simulink model "FCW_a1"  (Simulink 8.7)
settings: Solver=ode1  SolverMode=SingleTasking  StartTime=0.0  StopTime=500  FixedStep=0.001  RelTol=1e-3
(part 2 of 4)

== system FCW_a1/Veh_1_1/DriverModel ==
  note: Help
  VehicleInput : Inport
  Bus Creator37 : BusCreator  Inputs=10
  Bus Creator38 : BusCreator  Inputs=2
  Bus Creator39 : BusCreator  Inputs=2
  Bus Creator6 : BusCreator  Inputs=4
  Bus Selector : BusSelector  OutputSignals=Body_Out_Bus,Steer_Out_Bus,Power_Out_BUs,Brake_Out_Bus
  Bus Selector29 : BusSelector  OutputSignals=Chassi_States.q0,Chassi_States.q1,Chassi_States.q3,Chassi_States.u0,Chassi_States.u1,Chassi_States.u3,Wheel_LF.u1,Wheel_RF.u1,Wheel_LR.u1,Wheel_RR.u1
  Bus Selector30 : BusSelector  OutputSignals=Steer_Kinematics.str_sus_f,Steer_Kinematics.str_sus_r
  Bus Selector31 : BusSelector  OutputSignals=Powertrain_Output.av_eng,Powertrain_Output.aa_eng
  Bus Selector32 : BusSelector  OutputSignals=Brake_Output.turn_off
  Driver : Subsystem
  DriverOut : Outport
  wires:
  Bus Creator6/1 -> DriverOut/1  "Driver_Bus"
  Bus Creator39/1 -> Driver/3(Engine Input)
  Bus Selector31/2 -> Bus Creator39/2  "<aa_eng>"
  Bus Selector31/1 -> Bus Creator39/1  "<av_eng>"
  Bus Selector/3 -> Bus Selector31/1  "<Power_Out_BUs>"
  Bus Selector32/1 -> Driver/4(Brake Input)  "<turn_off>"
  Bus Creator38/1 -> Driver/2(Steer Input)
  Bus Selector30/2 -> Bus Creator38/2  "<str_sus_r>"
  Bus Selector30/1 -> Bus Creator38/1  "<str_sus_f>"
  Bus Selector/2 -> Bus Selector30/1  "<Steer_Out_Bus>"
  Bus Selector29/10 -> Bus Creator37/10  "<u1>"
  Bus Selector29/9 -> Bus Creator37/9  "<u1>"
  Bus Selector29/8 -> Bus Creator37/8  "<u1>"
  Bus Selector29/7 -> Bus Creator37/7  "<u1>"
  Bus Selector29/6 -> Bus Creator37/6  "<u3>"
  Bus Selector29/5 -> Bus Creator37/5  "<u1>"
  Bus Selector29/4 -> Bus Creator37/4  "<u0>"
  Bus Selector29/3 -> Bus Creator37/3  "<q3>"
  Bus Selector29/2 -> Bus Creator37/2  "<q1>"
  Bus Selector29/1 -> Bus Creator37/1  "<q0>"
  Bus Creator37/1 -> Driver/1(Body Input)
  Bus Selector/1 -> Bus Selector29/1  "<Body_Out_Bus>"
  Driver/4(Driver_Brake) -> Bus Creator6/4
  Driver/3(Driver_Powertrain) -> Bus Creator6/3
  Driver/2(Driver_Steer) -> Bus Creator6/2
  Driver/1(Driver_States) -> Bus Creator6/1
  VehicleInput/1 -> Bus Selector/1
  Bus Selector/4 -> Bus Selector32/1  "<Brake_Out_Bus>"

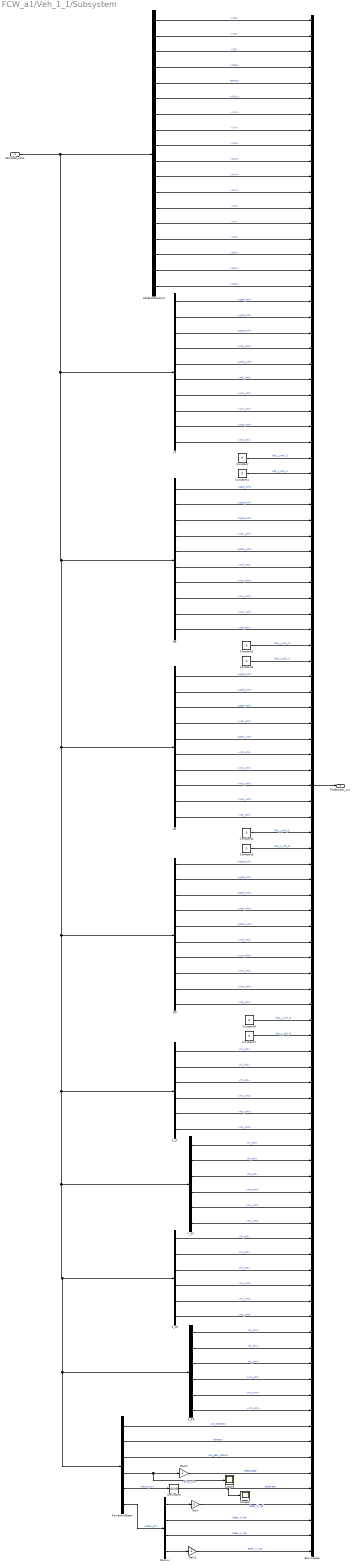
== system FCW_a1/Veh_1_1/Subsystem ==
  VehicleDynOut : Inport
  Bus Creator : BusCreator  Inputs=99
  Constant{,1..7} (8 alike) : Constant  Value=0
  Demux : Demux
  Derivative : Derivative
  F_LF : BusSelector  Tag=PanoSim_System  OutputSignals=Body_Out_Bus.Wheel_LF.fx_whl,Body_Out_Bus.Wheel_LF.fy_whl,Body_Out_Bus.Wheel_LF.fz_whl,Body_Out_Bus.Wheel_LF.mx_whl,Body_Out_Bus.Wheel_LF.my_whl,Body_Out_Bus.Wheel_LF.mz_whl
  F_LR : BusSelector  Tag=PanoSim_System  OutputSignals=Body_Out_Bus.Wheel_LR.fx_whl,Body_Out_Bus.Wheel_LR.fy_whl,Body_Out_Bus.Wheel_LR.fz_whl,Body_Out_Bus.Wheel_LR.mx_whl,Body_Out_Bus.Wheel_LR.my_whl,Body_Out_Bus.Wheel_LR.mz_whl
  F_RF : BusSelector  Tag=PanoSim_System  OutputSignals=Body_Out_Bus.Wheel_RF.fx_whl,Body_Out_Bus.Wheel_RF.fy_whl,Body_Out_Bus.Wheel_RF.fz_whl,Body_Out_Bus.Wheel_RF.mx_whl,Body_Out_Bus.Wheel_RF.my_whl,Body_Out_Bus.Wheel_RF.mz_whl
  F_RR : BusSelector  Tag=PanoSim_System  OutputSignals=Body_Out_Bus.Wheel_RR.fx_whl,Body_Out_Bus.Wheel_RR.fy_whl,Body_Out_Bus.Wheel_RR.fz_whl,Body_Out_Bus.Wheel_RR.mx_whl,Body_Out_Bus.Wheel_RR.my_whl,Body_Out_Bus.Wheel_RR.mz_whl
  Gain : Gain  Gain=-1
  Gain1 : Gain  Gain=-1
  Gain2 : Gain
  LF : BusSelector  Tag=PanoSim_System  OutputSignals=BodyKin_Wheel_Out_Bus.bodykin_whl_out_lf.xgnd_whl,BodyKin_Wheel_Out_Bus.bodykin_whl_out_lf.ygnd_whl,BodyKin_Wheel_Out_Bus.bodykin_whl_out_lf.zgnd_whl,BodyKin_Wheel_Out_Bus.bodykin_whl_out_lf.yaw_whl,BodyKin_Wheel_Out_Bus.bodykin_whl_out_lf.pitch_whl,BodyKin_Wheel_Out_Bus.bodykin_whl_out_lf.roll_whl,BodyKin_Wheel_Out_Bus.bodykin_whl_out_lf.vwx_whl,BodyKin_Wheel_Out_Bus.bodykin_whl_out_lf.vwy_whl,BodyKin_Wheel_Out_Bus.bodykin_whl_out_lf.vwz_whl,BodyKin_Wheel_Out_Bus.bodykin_whl_out_lf.rot_whl
  LR : BusSelector  Tag=PanoSim_System  OutputSignals=BodyKin_Wheel_Out_Bus.bodykin_whl_out_lr.xgnd_whl,BodyKin_Wheel_Out_Bus.bodykin_whl_out_lr.ygnd_whl,BodyKin_Wheel_Out_Bus.bodykin_whl_out_lr.zgnd_whl,BodyKin_Wheel_Out_Bus.bodykin_whl_out_lr.yaw_whl,BodyKin_Wheel_Out_Bus.bodykin_whl_out_lr.pitch_whl,BodyKin_Wheel_Out_Bus.bodykin_whl_out_lr.roll_whl,BodyKin_Wheel_Out_Bus.bodykin_whl_out_lr.vwx_whl,BodyKin_Wheel_Out_Bus.bodykin_whl_out_lr.vwy_whl,BodyKin_Wheel_Out_Bus.bodykin_whl_out_lr.vwz_whl,BodyKin_Wheel_Out_Bus.bodykin_whl_out_lr.rot_whl
  PowerandSteer : BusSelector  Tag=PanoSim_System  OutputSignals=Power_Out_BUs.Powertrain_Output.pt_throttle,Brake_Out_Bus.Brake_Output.brake,Power_Out_BUs.Powertrain_Output.pt_gear_status,Steer_Out_Bus.Steer_Kinematics.strav_sw,Steer_Out_Bus.Steer_Kinematics.strav_sw,Steer_Out_Bus.Steer_Kinematics.steer_str
  RF : BusSelector  Tag=PanoSim_System  OutputSignals=BodyKin_Wheel_Out_Bus.bodykin_whl_out_rf.xgnd_whl,BodyKin_Wheel_Out_Bus.bodykin_whl_out_rf.ygnd_whl,BodyKin_Wheel_Out_Bus.bodykin_whl_out_rf.zgnd_whl,BodyKin_Wheel_Out_Bus.bodykin_whl_out_rf.yaw_whl,BodyKin_Wheel_Out_Bus.bodykin_whl_out_rf.pitch_whl,BodyKin_Wheel_Out_Bus.bodykin_whl_out_rf.roll_whl,BodyKin_Wheel_Out_Bus.bodykin_whl_out_rf.vwx_whl,BodyKin_Wheel_Out_Bus.bodykin_whl_out_rf.vwy_whl,BodyKin_Wheel_Out_Bus.bodykin_whl_out_rf.vwz_whl,BodyKin_Wheel_Out_Bus.bodykin_whl_out_rf.rot_whl
  RR : BusSelector  Tag=PanoSim_System  OutputSignals=BodyKin_Wheel_Out_Bus.bodykin_whl_out_rr.xgnd_whl,BodyKin_Wheel_Out_Bus.bodykin_whl_out_rr.ygnd_whl,BodyKin_Wheel_Out_Bus.bodykin_whl_out_rr.zgnd_whl,BodyKin_Wheel_Out_Bus.bodykin_whl_out_rr.yaw_whl,BodyKin_Wheel_Out_Bus.bodykin_whl_out_rr.pitch_whl,BodyKin_Wheel_Out_Bus.bodykin_whl_out_rr.roll_whl,BodyKin_Wheel_Out_Bus.bodykin_whl_out_rr.vwx_whl,BodyKin_Wheel_Out_Bus.bodykin_whl_out_rr.vwy_whl,BodyKin_Wheel_Out_Bus.bodykin_whl_out_rr.vwz_whl,BodyKin_Wheel_Out_Bus.bodykin_whl_out_rr.rot_whl
  Scope1 : Scope
  Scope6 : Scope
  VehBusSelector3 : BusSelector  Tag=PanoSim_System  OutputSignals=Body_Out_Bus.Chassis_Motion.XO,Body_Out_Bus.Chassis_Motion.YO,Body_Out_Bus.Chassis_Motion.ZO,Body_Out_Bus.Chassis_Motion.YAW,Body_Out_Bus.Chassis_Motion.PITCH,Body_Out_Bus.Chassis_Motion.ROLL,Body_Out_Bus.Chassis_Motion.VX,Body_Out_Bus.Chassis_Motion.VY,Body_Out_Bus.Chassis_Motion.VZ,Body_Out_Bus.Chassis_Motion.AVZ,Body_Out_Bus.Chassis_Motion.AVY,Body_Out_Bus.Chassis_Motion.AVX,Body_Out_Bus.Chassis_Motion.AX,Body_Out_Bus.Chassis_Motion.AY,Body_Out_Bus.Chassis_Motion.AZ,Body_Out_Bus.Chassis_Motion.AAX,Body_Out_Bus.Chassis_Motion.AAY,Body_Out_Bus.Chassis_Motion.AAZ
  PlotBuilder_out : Outport
  wires:
  Bus Creator/1 -> PlotBuilder_out/1
  PowerandSteer/6 -> Demux/1  "<steer_str>"
  LF/9 -> Bus Creator/27  "<vwz_whl>"
  LF/6 -> Bus Creator/24  "<roll_whl>"
  F_LR/6 -> Bus Creator/84  "<mz_whl>"
  F_LR/5 -> Bus Creator/83  "<my_whl>"
  F_LR/3 -> Bus Creator/81  "<fz_whl>"
  Constant4/1 -> Bus Creator/53  "Rot_y_whl_l2"
  RF/9 -> Bus Creator/39  "<vwz_whl>"
  F_LR/2 -> Bus Creator/80  "<fy_whl>"
  RF/4 -> Bus Creator/34  "<yaw_whl>"
  RF/5 -> Bus Creator/35  "<pitch_whl>"
  LR/10 -> Bus Creator/52  "<rot_whl>"
  LR/9 -> Bus Creator/51  "<vwz_whl>"
  LR/8 -> Bus Creator/50  "<vwy_whl>"
  LR/6 -> Bus Creator/48  "<roll_whl>"
  LR/7 -> Bus Creator/49  "<vwx_whl>"
  LR/4 -> Bus Creator/46  "<yaw_whl>"
  LR/5 -> Bus Creator/47  "<pitch_whl>"
  LR/1 -> Bus Creator/43  "<xgnd_whl>"
  LR/2 -> Bus Creator/44  "<ygnd_whl>"
  PowerandSteer/5 -> Derivative/1  "<strav_sw>"
  VehBusSelector3/18 -> Bus Creator/18  "<AAZ>"
  RF/3 -> Bus Creator/33  "<zgnd_whl>"
  VehBusSelector3/17 -> Bus Creator/17  "<AAY>"
  Demux/4 -> Gain1/1
  VehBusSelector3/16 -> Bus Creator/16  "<AAX>"
  VehBusSelector3/14 -> Bus Creator/14  "<AY>"
  VehBusSelector3/13 -> Bus Creator/13  "<AX>"
  LF/4 -> Bus Creator/22  "<yaw_whl>"
  F_LF/6 -> Bus Creator/72  "<mz_whl>"
  F_LF/5 -> Bus Creator/71  "<my_whl>"
  F_LF/4 -> Bus Creator/70  "<mx_whl>"
  F_LF/3 -> Bus Creator/69  "<fz_whl>"
  F_LF/2 -> Bus Creator/68  "<fy_whl>"
  F_LF/1 -> Bus Creator/67  "<fx_whl>"
  RF/7 -> Bus Creator/37  "<vwx_whl>"
  RF/6 -> Bus Creator/36  "<roll_whl>"
  Constant1/1 -> Bus Creator/30  "Rot_z_whl_l1"
  F_RR/5 -> Bus Creator/89  "<my_whl>"
  RF/10 -> Bus Creator/40  "<rot_whl>"
  F_LR/1 -> Bus Creator/79  "<fx_whl>"
  F_RR/2 -> Bus Creator/86  "<fy_whl>"
  F_RR/1 -> Bus Creator/85  "<fx_whl>"
  Constant/1 -> Bus Creator/29  "Rot_y_whl_l1"
  F_RR/4 -> Bus Creator/88  "<mx_whl>"
  VehBusSelector3/5 -> Bus Creator/5  "<PITCH>"
  LF/8 -> Bus Creator/26  "<vwy_whl>"
  RR/4 -> Bus Creator/58  "<yaw_whl>"
  F_RR/3 -> Bus Creator/87  "<fz_whl>"
  VehBusSelector3/8 -> Bus Creator/8  "<VY>"
  RR/3 -> Bus Creator/57  "<zgnd_whl>"
  VehBusSelector3/11 -> Bus Creator/11  "<AVY>"
  RR/2 -> Bus Creator/56  "<ygnd_whl>"
  PowerandSteer/4 -> Gain2/1, Scope6/1  "<strav_sw>"
  Demux/3 -> Bus Creator/98  "Steer_lr_rad"
  F_RF/2 -> Bus Creator/74  "<fy_whl>"
  RR/1 -> Bus Creator/55  "<xgnd_whl>"
  F_RR/6 -> Bus Creator/90  "<mz_whl>"
  RR/10 -> Bus Creator/64  "<rot_whl>"
  Gain1/1 -> Bus Creator/99  "Steer_rr_rad"
  RR/7 -> Bus Creator/61  "<vwx_whl>"
  Constant7/1 -> Bus Creator/66  "Rot_z_whl_r2"
  F_RF/4 -> Bus Creator/76  "<mx_whl>"
  VehBusSelector3/6 -> Bus Creator/6  "<ROLL>"
  Constant3/1 -> Bus Creator/42  "Rot_z_whl_r1"
  Constant2/1 -> Bus Creator/41  "Rot_y_whl_r1"
  RR/9 -> Bus Creator/63  "<vwz_whl>"
  VehBusSelector3/1 -> Bus Creator/1  "<XO>"
  RR/8 -> Bus Creator/62  "<vwy_whl>"
  Constant6/1 -> Bus Creator/65  "Rot_y_whl_r2"
  VehBusSelector3/9 -> Bus Creator/9  "<VZ>"
  RR/6 -> Bus Creator/60  "<roll_whl>"
  Derivative/1 -> Scope1/1, Bus Creator/95  "Steerrate"
  VehBusSelector3/3 -> Bus Creator/3  "<ZO>"
  RF/1 -> Bus Creator/31  "<xgnd_whl>"
  RF/8 -> Bus Creator/38  "<vwy_whl>"
  Constant5/1 -> Bus Creator/54  "Rot_z_whl_l2"
  VehBusSelector3/10 -> Bus Creator/10  "<AVZ>"
  LF/1 -> Bus Creator/19  "<xgnd_whl>"
  F_RF/5 -> Bus Creator/77  "<my_whl>"
  PowerandSteer/2 -> Bus Creator/92  "<brake>"
  Gain2/1 -> Bus Creator/94  "Steerangle"
  VehicleDynOut/1 -> VehBusSelector3/1, LF/1, RF/1, LR/1, RR/1, F_LF/1, F_RF/1, F_LR/1, F_RR/1, PowerandSteer/1
  F_RF/6 -> Bus Creator/78  "<mz_whl>"
  VehBusSelector3/2 -> Bus Creator/2  "<YO>"
  Demux/2 -> Bus Creator/97  "Steer_rf_rad"
  LF/2 -> Bus Creator/20  "<ygnd_whl>"
  LF/7 -> Bus Creator/25  "<vwx_whl>"
  PowerandSteer/3 -> Bus Creator/93  "<pt_gear_status>"
  VehBusSelector3/7 -> Bus Creator/7  "<VX>"
  LR/3 -> Bus Creator/45  "<zgnd_whl>"
  VehBusSelector3/15 -> Bus Creator/15  "<AZ>"
  VehBusSelector3/4 -> Bus Creator/4  "<YAW>"
  Gain/1 -> Bus Creator/96  "Steer_lf_rad"
  RR/5 -> Bus Creator/59  "<pitch_whl>"
  PowerandSteer/1 -> Bus Creator/91  "<pt_throttle>"
  LF/5 -> Bus Creator/23  "<pitch_whl>"
  F_LR/4 -> Bus Creator/82  "<mx_whl>"
  F_RF/3 -> Bus Creator/75  "<fz_whl>"
  LF/10 -> Bus Creator/28  "<rot_whl>"
  RF/2 -> Bus Creator/32  "<ygnd_whl>"
  Demux/1 -> Gain/1
  VehBusSelector3/12 -> Bus Creator/12  "<AVX>"
  LF/3 -> Bus Creator/21  "<zgnd_whl>"
  F_RF/1 -> Bus Creator/73  "<fx_whl>"

== system FCW_a1/Veh_1_1/Veh_1_1_Sensors ==
  note: Help
  note: Help
  In1 : Inport
  OBU_BSM : Subsystem  Tag=PanoSim_System
      mask Display: image(imread('V2X.png'));
  SensorBus : BusCreator  Inputs=1
  Out1 : Outport
  wires:
  SensorBus/1 -> Out1/1
  In1/1 -> OBU_BSM/1(In1)
  OBU_BSM/1(Out1) -> SensorBus/1  "OBU_BSM_Out"

== system FCW_a1/Veh_1/ComplexVehicleModel/Aerodynamics ==
  Body Input : Inport
  Aerodynamics Model : S-Function  FunctionName=panoAerodynamics_sfun  Parameters='2f869580-59bc-4052-87af-10578d1ae191'  SFunctionDeploymentMode=off  EnableBusSupport=off
  Chassis States : Subsystem
  Memory : Memory
  Aerodymatics Out : Outport
  wires:
  Body Input/1 -> Memory/1
  Aerodynamics Model/1 -> Chassis States/1(In1)
  Chassis States/1(Out1) -> Aerodymatics Out/1  "Aerodynamics_Output"
  Memory/1 -> Aerodynamics Model/1

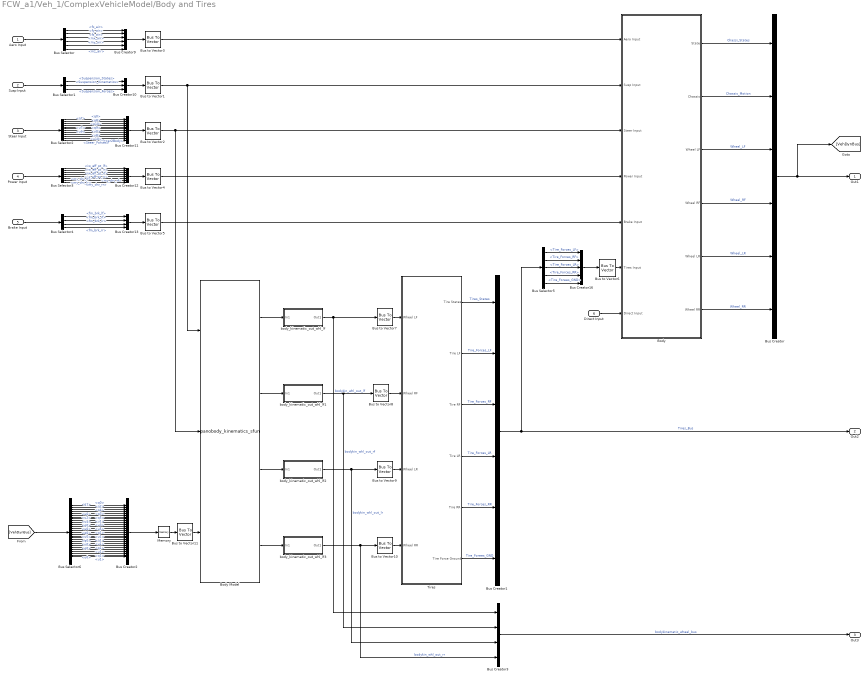
== system FCW_a1/Veh_1/ComplexVehicleModel/Body and Tires ==
  Aero Input : Inport
  Susp Input : Inport  Port=2
  Steer Input : Inport  Port=3
  Power Input : Inport  Port=4
  Brake Input : Inport  Port=5
  Direct Input : Inport  Port=6
  Body : Subsystem
  Body Model : S-Function  FunctionName=panobody_kinematics_sfun  Parameters='2f869580-59bc-4052-87af-10578d1ae191'  SFunctionDeploymentMode=off  EnableBusSupport=off
  Bus Creator : BusCreator  Inputs=6
  Bus Creator1 : BusCreator  Inputs=6
  Bus Creator10 : BusCreator  Inputs=3
  Bus Creator11 : BusCreator  Inputs=12
  Bus Creator12 : BusCreator  Inputs=8
  Bus Creator13 : BusCreator  Inputs=4
  Bus Creator16 : BusCreator  Inputs=5
  Bus Creator2 : BusCreator  Inputs=28
  Bus Creator3 : BusCreator  Inputs=4
  Bus Creator9 : BusCreator  Inputs=6
  Bus Selector : BusSelector  OutputSignals=Aerodynamics_Output.fx_air,Aerodynamics_Output.fy_air,Aerodynamics_Output.fz_air,Aerodynamics_Output.mx_air,Aerodynamics_Output.my_air,Aerodynamics_Output.mz_air
  Bus Selector1 : BusSelector  OutputSignals=Suspension_States,Suspension_Kinematics,Suspension_Forces
  Bus Selector2 : BusSelector  OutputSignals=Steer_States.q0,Steer_States.q7,Steer_States.q8,Steer_States.q9,Steer_States.q10,Steer_States.u0,Steer_States.u7,Steer_States.u8,Steer_States.u9,Steer_States.u10,Steer2Body,Steer_Forces
  Bus Selector3 : BusSelector  OutputSignals=Powertrain_Output.iw_eff_pt_lf,Powertrain_Output.iw_eff_pt_rf,Powertrain_Output.iw_eff_pt_lr,Powertrain_Output.iw_eff_pt_rr,Powertrain_Output.my_drv_lf,Powertrain_Output.my_drv_rf,Powertrain_Output.my_drv_lr,Powertrain_Output.my_drv_rr
  Bus Selector4 : BusSelector  OutputSignals=Brake_Output.fm_brk_lf,Brake_Output.fm_brk_rf,Brake_Output.fm_brk_lr,Brake_Output.fm_brk_rr
  Bus Selector5 : BusSelector  OutputSignals=Tire_Forces_LF,Tire_Forces_RF,Tire_Forces_LR,Tire_Forces_RR,Tire_Forees_GND
  Bus Selector6 : BusSelector  OutputSignals=Chassi_States.q0,Chassi_States.q1,Chassi_States.q2,Chassi_States.q3,Chassi_States.q4,Chassi_States.q5,Chassi_States.u0,Chassi_States.u1,Chassi_States.u2,Chassi_States.u3,Chassi_States.u4,Chassi_States.u5,Wheel_LF.q0,Wheel_LF.q1,Wheel_LF.u0,Wheel_LF.u1,Wheel_RF.q0,Wheel_RF.q1,Wheel_RF.u0,Wheel_RF.u1,Wheel_LR.q0,Wheel_LR.q1,Wheel_LR.u0,Wheel_LR.u1,Wheel_RR.q0,Wheel_RR.q1,Wheel_RR.u0,Wheel_RR.u1
  Bus to Vector{1..11} (11 alike) : BusToVector
  Memory : Memory
  Tires : Subsystem
  body_kinematic_out_whl_lf : Subsystem
  body_kinematic_out_whl_lf1 : Subsystem
  body_kinematic_out_whl_lf2 : Subsystem
  body_kinematic_out_whl_lf3 : Subsystem
  Out1 : Outport
  Out2 : Outport  Port=2
  Out3 : Outport  Port=3
  wires:
  Bus Selector5/5 -> Bus Creator16/5  "<Tire_Forees_GND>"
  Tires/6(Tire Force Ground) -> Bus Creator1/6  "Tire_Forees_GND"
  Aero Input/1 -> Bus Selector/1
  Susp Input/1 -> Bus Selector1/1
  Body/1(State) -> Bus Creator/1  "Chassi_States"
  Body/2(Chassis) -> Bus Creator/2  "Chassis_Motion"
  Body/3(Wheel LF) -> Bus Creator/3  "Wheel_LF"
  Body/4(Wheel RF) -> Bus Creator/4  "Wheel_RF"
  Body/5(Wheel LR) -> Bus Creator/5  "Wheel_LR"
  Body/6(Wheel RR) -> Bus Creator/6  "Wheel_RR"
  Bus Selector/1 -> Bus Creator9/1  "<fx_air>"
  Bus Selector/2 -> Bus Creator9/2  "<fy_air>"
  Bus Selector/3 -> Bus Creator9/3  "<fz_air>"
  Bus Selector/4 -> Bus Creator9/4  "<mx_air>"
  Bus Selector/5 -> Bus Creator9/5  "<my_air>"
  Bus Selector/6 -> Bus Creator9/6  "<mz_air>"
  Bus Selector1/1 -> Bus Creator10/1  "<Suspension_States>"
  Bus Selector1/2 -> Bus Creator10/2  "<Suspension_Kinematics>"
  Bus Selector3/1 -> Bus Creator12/1  "<iw_eff_pt_lf>"
  Bus Selector3/2 -> Bus Creator12/2  "<iw_eff_pt_rf>"
  Bus Selector3/3 -> Bus Creator12/3  "<iw_eff_pt_lr>"
  Bus Selector3/4 -> Bus Creator12/4  "<iw_eff_pt_rr>"
  Bus Selector4/1 -> Bus Creator13/1  "<fm_brk_lf>"
  Bus Selector4/2 -> Bus Creator13/2  "<fm_brk_rf>"
  Bus Selector4/3 -> Bus Creator13/3  "<fm_brk_lr>"
  Bus Selector4/4 -> Bus Creator13/4  "<fm_brk_rr>"
  Bus Selector5/1 -> Bus Creator16/1  "<Tire_Forces_LF>"
  Bus Selector5/2 -> Bus Creator16/2  "<Tire_Forces_RF>"
  Bus Selector5/3 -> Bus Creator16/3  "<Tire_Forces_LR>"
  Bus Selector5/4 -> Bus Creator16/4  "<Tire_Forces_RR>"
  Bus Creator16/1 -> Bus to Vector6/1
  Bus Selector2/1 -> Bus Creator11/1  "<q0>"
  Bus Selector2/2 -> Bus Creator11/2  "<q7>"
  Bus Selector2/3 -> Bus Creator11/3  "<q8>"
  Bus Selector2/4 -> Bus Creator11/4  "<q9>"
  Bus Selector2/5 -> Bus Creator11/5  "<q10>"
  Bus Selector2/6 -> Bus Creator11/6  "<u0>"
  Bus Selector2/7 -> Bus Creator11/7  "<u7>"
  Bus Selector2/8 -> Bus Creator11/8  "<u8>"
  Bus Selector2/9 -> Bus Creator11/9  "<u9>"
  Bus Selector2/10 -> Bus Creator11/10  "<u10>"
  Bus Selector2/11 -> Bus Creator11/11  "<Steer2Body>"
  Bus Selector2/12 -> Bus Creator11/12  "<Steer_Forces>"
  Bus Creator/1 -> Out1/1, [VehDynBus]
  Tires/1(Tire States) -> Bus Creator1/1  "Tires_States"
  Tires/2(Tire LF) -> Bus Creator1/2  "Tire_Forces_LF"
  Tires/3(Tire RF) -> Bus Creator1/3  "Tire_Forces_RF"
  Tires/4(Tire LR) -> Bus Creator1/4  "Tire_Forces_LR"
  Tires/5(Tire RR) -> Bus Creator1/5  "Tire_Forces_RR"
  Bus Creator1/1 -> Bus Selector5/1, Out2/1  "Tires_Bus"
  Power Input/1 -> Bus Selector3/1
  Direct Input/1 -> Body/7(Direct Input)
  Brake Input/1 -> Bus Selector4/1
  Body Model/1 -> body_kinematic_out_whl_lf/1(In1)
  Body Model/2 -> body_kinematic_out_whl_lf1/1(In1)
  Body Model/3 -> body_kinematic_out_whl_lf2/1(In1)
  Body Model/4 -> body_kinematic_out_whl_lf3/1(In1)
  Steer Input/1 -> Bus Selector2/1
  Bus Selector1/3 -> Bus Creator10/3  "<Suspension_Forces>"
  Bus Selector3/5 -> Bus Creator12/5  "<my_drv_lf>"
  Bus Selector3/6 -> Bus Creator12/6  "<my_drv_rf>"
  Bus Selector3/7 -> Bus Creator12/7  "<my_drv_lr>"
  Bus Selector3/8 -> Bus Creator12/8  "<my_drv_rr>"
  Bus Creator10/1 -> Bus to Vector1/1
  [VehDynBus] -> Bus Selector6/1
  Bus Selector6/1 -> Bus Creator2/1  "<q0>"
  Bus Selector6/2 -> Bus Creator2/2  "<q1>"
  Bus Selector6/3 -> Bus Creator2/3  "<q2>"
  Bus Selector6/4 -> Bus Creator2/4  "<q3>"
  Bus Selector6/5 -> Bus Creator2/5  "<q4>"
  Bus Selector6/6 -> Bus Creator2/6  "<q5>"
  Bus Selector6/7 -> Bus Creator2/7  "<u0>"
  Bus Selector6/8 -> Bus Creator2/8  "<u1>"
  Bus Selector6/9 -> Bus Creator2/9  "<u2>"
  Bus Selector6/10 -> Bus Creator2/10  "<u3>"
  Bus Selector6/11 -> Bus Creator2/11  "<u4>"
  Bus Selector6/12 -> Bus Creator2/12  "<u5>"
  Bus Selector6/13 -> Bus Creator2/13  "<q0>"
  Bus Selector6/14 -> Bus Creator2/14  "<q1>"
  Bus Selector6/15 -> Bus Creator2/15  "<u0>"
  Bus Selector6/16 -> Bus Creator2/16  "<u1>"
  Bus Selector6/17 -> Bus Creator2/17  "<q0>"
  Bus Selector6/18 -> Bus Creator2/18  "<q1>"
  Bus Selector6/19 -> Bus Creator2/19  "<u0>"
  Bus Selector6/20 -> Bus Creator2/20  "<u1>"
  Bus Selector6/21 -> Bus Creator2/21  "<q0>"
  Bus Selector6/22 -> Bus Creator2/22  "<q1>"
  Bus Selector6/23 -> Bus Creator2/23  "<u0>"
  Bus Selector6/24 -> Bus Creator2/24  "<u1>"
  Bus Selector6/25 -> Bus Creator2/25  "<q0>"
  Bus Selector6/26 -> Bus Creator2/26  "<q1>"
  Bus Selector6/27 -> Bus Creator2/27  "<u0>"
  Bus Selector6/28 -> Bus Creator2/28  "<u1>"
  Bus Creator2/1 -> Memory/1
  Memory/1 -> Bus to Vector11/1
  Bus Creator11/1 -> Bus to Vector2/1
  Bus Creator9/1 -> Bus to Vector3/1
  Bus Creator12/1 -> Bus to Vector4/1
  Bus Creator13/1 -> Bus to Vector5/1
  body_kinematic_out_whl_lf/1(Out1) -> Bus to Vector7/1, Bus Creator3/1  "bodykin_whl_out_lf"
  body_kinematic_out_whl_lf1/1(Out1) -> Bus to Vector8/1, Bus Creator3/2  "bodykin_whl_out_rf"
  body_kinematic_out_whl_lf2/1(Out1) -> Bus to Vector9/1, Bus Creator3/3  "bodykin_whl_out_lr"
  body_kinematic_out_whl_lf3/1(Out1) -> Bus to Vector10/1, Bus Creator3/4  "bodykin_whl_out_rr"
  Bus Creator3/1 -> Out3/1  "bodykinematic_wheel_bus"
  Bus to Vector3/1 -> Body/1(Aero Input)
  Bus to Vector1/1 -> Body/2(Susp Input), Body Model/1
  Bus to Vector2/1 -> Body/3(Steer Input), Body Model/2
  Bus to Vector4/1 -> Body/4(Power Input)
  Bus to Vector5/1 -> Body/5(Brake Input)
  Bus to Vector6/1 -> Body/6(Tires Input)
  Bus to Vector7/1 -> Tires/1(Wheel LF)
  Bus to Vector8/1 -> Tires/2(Wheel RF)
  Bus to Vector9/1 -> Tires/3(Wheel LR)
  Bus to Vector10/1 -> Tires/4(Wheel RR)
  Bus to Vector11/1 -> Body Model/3

== system FCW_a1/Veh_1/ComplexVehicleModel/Brake ==
  Body Input : Inport
  Driver Input : Inport  Port=2
  Inertia Wheel : Inport  Port=3
  Fz Wheel : Inport  Port=4
  Direct Input : Inport  Port=5
  Brake Model : S-Function  FunctionName=panoBrake_sfun  Parameters='2f869580-59bc-4052-87af-10578d1ae191'  SFunctionDeploymentMode=off  EnableBusSupport=off
  Brake States : Subsystem
  Memory : Memory
  SteerStates1 : Subsystem
  BrakeStates : Outport
  BrakeOutput : Outport  Port=2
  wires:
  Direct Input/1 -> Brake Model/5
  Brake Model/1 -> Brake States/1(In1)
  Brake Model/2 -> SteerStates1/1(In1)
  Body Input/1 -> Memory/1
  Driver Input/1 -> Brake Model/2
  Inertia Wheel/1 -> Brake Model/3
  Fz Wheel/1 -> Brake Model/4
  Brake States/1(Out1) -> BrakeStates/1
  SteerStates1/1(Out1) -> BrakeOutput/1
  Memory/1 -> Brake Model/1

== system FCW_a1/Veh_1/ComplexVehicleModel/Powertrain ==
  Body Input : Inport
  Throttle : Inport  Port=2
  TransMode : Inport  Port=3
  Gear : Inport  Port=4
  BrakeSignal : Inport  Port=5
  Memory : Memory
  Powertrain Model : S-Function  FunctionName=panoPowertrain_sfun  Parameters='2f869580-59bc-4052-87af-10578d1ae191'  SFunctionDeploymentMode=off  EnableBusSupport=off
  PowertrainOut : Subsystem
  PowertrainStates : Subsystem
  Powertrain States : Outport
  Powertrain Output : Outport  Port=2
  wires:
  BrakeSignal/1 -> Powertrain Model/5
  Gear/1 -> Powertrain Model/4
  TransMode/1 -> Powertrain Model/3
  Throttle/1 -> Powertrain Model/2
  Powertrain Model/1 -> PowertrainStates/1(In1)
  PowertrainStates/1(Out1) -> Powertrain States/1
  PowertrainOut/1(Out1) -> Powertrain Output/1
  Powertrain Model/2 -> PowertrainOut/1(In1)
  Memory/1 -> Powertrain Model/1
  Body Input/1 -> Memory/1

== system FCW_a1/Veh_1/ComplexVehicleModel/Steer ==
  Body Input : Inport
  Steer Angle : Inport  Port=2
  Suspension Input : Inport  Port=3
  Tire Input : Inport  Port=4
  Direct Steer : Inport  Port=5
  Memory : Memory
  Memory1 : Memory
  SteerForces : Subsystem
  SteerKinemateics : Subsystem
  SteerStates : Subsystem
  SteerToBody : Subsystem
  Steering Model : S-Function  FunctionName=panoSteer_sfun  Parameters='2f869580-59bc-4052-87af-10578d1ae191'  SFunctionDeploymentMode=off  EnableBusSupport=off
  Steer States : Outport
  Steer Kinematiocs : Outport  Port=2
  Steer2Body : Outport  Port=3
  Steer Forces : Outport  Port=4
  wires:
  Direct Steer/1 -> Steering Model/5
  Body Input/1 -> Memory/1
  Suspension Input/1 -> Steering Model/3
  Tire Input/1 -> Memory1/1
  Steer Angle/1 -> Steering Model/2
  Steering Model/1 -> SteerStates/1(In1)
  SteerStates/1(Out1) -> Steer States/1  "Steer_States"
  SteerKinemateics/1(Out1) -> Steer Kinematiocs/1  "Steer_Kinematics"
  SteerToBody/1(Out1) -> Steer2Body/1  "SteertoBody"
  SteerForces/1(Out1) -> Steer Forces/1  "Steer_Forces"
  Steering Model/2 -> SteerKinemateics/1(In1)
  Steering Model/3 -> SteerToBody/1(In1)
  Steering Model/4 -> SteerForces/1(In1)
  Memory/1 -> Steering Model/1
  Memory1/1 -> Steering Model/4

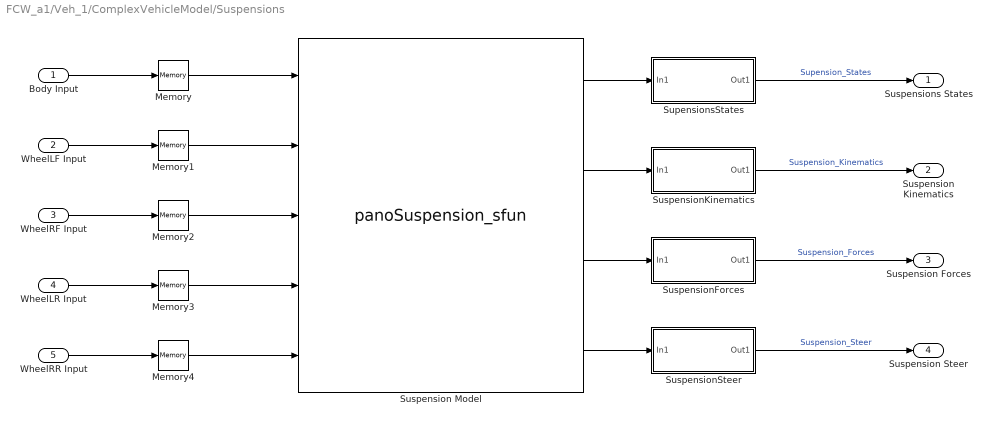
== system FCW_a1/Veh_1/ComplexVehicleModel/Suspensions ==
  Body Input : Inport
  WheelLF Input : Inport  Port=2
  WheelRF Input : Inport  Port=3
  WheelLR Input : Inport  Port=4
  WheelRR Input : Inport  Port=5
  Memory{,1..4} (5 alike) : Memory
  SupensionsStates : Subsystem
  Suspension Model : S-Function  FunctionName=panoSuspension_sfun  Parameters='2f869580-59bc-4052-87af-10578d1ae191'  SFunctionDeploymentMode=off  EnableBusSupport=off
  SuspensionForces : Subsystem
  SuspensionKinematics : Subsystem
  SuspensionSteer : Subsystem
  Suspensions States : Outport
  Suspension Kinematics : Outport  Port=2
  Suspension Forces : Outport  Port=3
  Suspension Steer : Outport  Port=4
  wires:
  Body Input/1 -> Memory/1
  WheelLF Input/1 -> Memory1/1
  WheelRF Input/1 -> Memory2/1
  WheelLR Input/1 -> Memory3/1
  WheelRR Input/1 -> Memory4/1
  Suspension Model/1 -> SupensionsStates/1(In1)
  SupensionsStates/1(Out1) -> Suspensions States/1  "Supension_States"
  SuspensionKinematics/1(Out1) -> Suspension Kinematics/1  "Suspension_Kinematics"
  SuspensionForces/1(Out1) -> Suspension Forces/1  "Suspension_Forces"
  SuspensionSteer/1(Out1) -> Suspension Steer/1  "Suspension_Steer"
  Suspension Model/2 -> SuspensionKinematics/1(In1)
  Suspension Model/3 -> SuspensionForces/1(In1)
  Suspension Model/4 -> SuspensionSteer/1(In1)
  Memory/1 -> Suspension Model/1
  Memory1/1 -> Suspension Model/2
  Memory2/1 -> Suspension Model/3
  Memory3/1 -> Suspension Model/4
  Memory4/1 -> Suspension Model/5

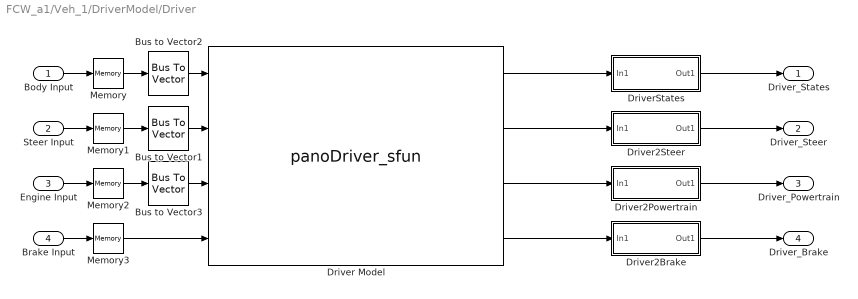
== system FCW_a1/Veh_1/DriverModel/Driver ==
  Body Input : Inport
  Steer Input : Inport  Port=2
  Engine Input : Inport  Port=3
  Brake Input : Inport  Port=4
  Bus to Vector1 : BusToVector
  Bus to Vector2 : BusToVector
  Bus to Vector3 : BusToVector
  Driver Model : S-Function  FunctionName=panoDriver_sfun  Parameters='2f869580-59bc-4052-87af-10578d1ae191'  SFunctionDeploymentMode=off  EnableBusSupport=off
  Driver2Brake : Subsystem
  Driver2Powertrain : Subsystem
  Driver2Steer : Subsystem
  DriverStates : Subsystem
  Memory{,1..3} (4 alike) : Memory
  Driver_States : Outport
  Driver_Steer : Outport  Port=2
  Driver_Powertrain : Outport  Port=3
  Driver_Brake : Outport  Port=4
  wires:
  Memory3/1 -> Driver Model/4
  Memory2/1 -> Bus to Vector3/1
  Memory1/1 -> Bus to Vector1/1
  Memory/1 -> Bus to Vector2/1
  Body Input/1 -> Memory/1
  Steer Input/1 -> Memory1/1
  Driver2Powertrain/1(Out1) -> Driver_Powertrain/1
  Driver2Brake/1(Out1) -> Driver_Brake/1
  Driver Model/4 -> Driver2Brake/1(In1)
  Driver Model/3 -> Driver2Powertrain/1(In1)
  Driver2Steer/1(Out1) -> Driver_Steer/1
  Driver Model/2 -> Driver2Steer/1(In1)
  DriverStates/1(Out1) -> Driver_States/1
  Driver Model/1 -> DriverStates/1(In1)
  Engine Input/1 -> Memory2/1
  Brake Input/1 -> Memory3/1
  Bus to Vector2/1 -> Driver Model/1
  Bus to Vector1/1 -> Driver Model/2
  Bus to Vector3/1 -> Driver Model/3

== system FCW_a1/Veh_1/Veh_1_Sensors/OBU_BSM ==
  In1 : Inport
  Bus : BusCreator  Inputs=20
  GeneralSensor : S-Function  FunctionName=GeneralSensorModel  Parameters='PanoDataModel.Sensor.OBU.BSM.Output','1c1eb9b2-dd0f-4a4f-b3eb-ea51094d06de','pos.lat@f,pos.long@f,secMark@i,accuracy.pos@f,transmission@f,speed@f,heading@i,accelSet.long@f,accelSet.lat@f,accelSet.vert@f,accelSet.yaw@f,brakes.traction@i,brakes.abs@i,brakes.scs@i,size.width@f,size.length@f,vehicleClass.classification@i,safetyExt.events@i,safetyExt.lights@i','10.00','64'  SFunctionDeploymentMode=off  EnableBusSupport=off
  Out1 : Outport
  wires:
  GeneralSensor/1 -> Bus/1  "Width"
  In1/1 -> GeneralSensor/1
  Bus/1 -> Out1/1
  GeneralSensor/2 -> Bus/2  "pos.lat"
  GeneralSensor/3 -> Bus/3  "pos.long"
  GeneralSensor/4 -> Bus/4  "secMark"
  GeneralSensor/5 -> Bus/5  "accuracy.pos"
  GeneralSensor/6 -> Bus/6  "transmission"
  GeneralSensor/7 -> Bus/7  "speed"
  GeneralSensor/8 -> Bus/8  "heading"
  GeneralSensor/9 -> Bus/9  "accelSet.long"
  GeneralSensor/10 -> Bus/10  "accelSet.lat"
  GeneralSensor/11 -> Bus/11  "accelSet.vert"
  GeneralSensor/12 -> Bus/12  "accelSet.yaw"
  GeneralSensor/13 -> Bus/13  "brakes.traction"
  GeneralSensor/14 -> Bus/14  "brakes.abs"
  GeneralSensor/15 -> Bus/15  "brakes.scs"
  GeneralSensor/16 -> Bus/16  "size.width"
  GeneralSensor/17 -> Bus/17  "size.length"
  GeneralSensor/18 -> Bus/18  "vehicleClass.classification"
  GeneralSensor/19 -> Bus/19  "safetyExt.events"
  GeneralSensor/20 -> Bus/20  "safetyExt.lights"

== system FCW_a1/Veh_1_1/ComplexVehicleModel/Aerodynamics ==
  Body Input : Inport
  Aerodynamics Model : S-Function  FunctionName=panoAerodynamics_sfun  Parameters='5aa55ff1-4ffb-47ef-b8cb-7b2ffdefc837'  SFunctionDeploymentMode=off  EnableBusSupport=off
  Chassis States : Subsystem
  Memory : Memory
  Aerodymatics Out : Outport
  wires:
  Body Input/1 -> Memory/1
  Aerodynamics Model/1 -> Chassis States/1(In1)
  Chassis States/1(Out1) -> Aerodymatics Out/1  "Aerodynamics_Output"
  Memory/1 -> Aerodynamics Model/1

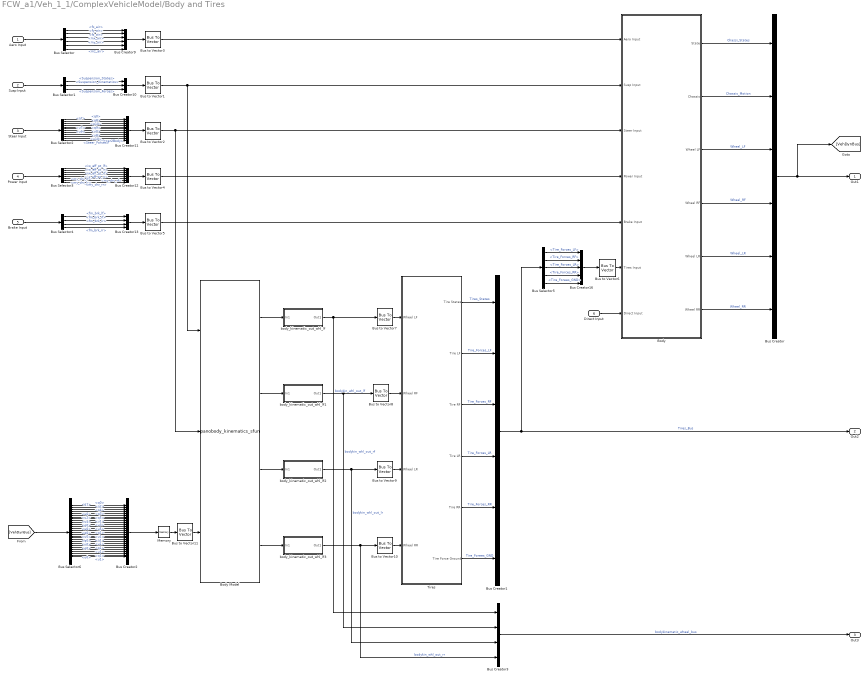
== system FCW_a1/Veh_1_1/ComplexVehicleModel/Body and Tires ==
  Aero Input : Inport
  Susp Input : Inport  Port=2
  Steer Input : Inport  Port=3
  Power Input : Inport  Port=4
  Brake Input : Inport  Port=5
  Direct Input : Inport  Port=6
  Body : Subsystem
  Body Model : S-Function  FunctionName=panobody_kinematics_sfun  Parameters='5aa55ff1-4ffb-47ef-b8cb-7b2ffdefc837'  SFunctionDeploymentMode=off  EnableBusSupport=off
  Bus Creator : BusCreator  Inputs=6
  Bus Creator1 : BusCreator  Inputs=6
  Bus Creator10 : BusCreator  Inputs=3
  Bus Creator11 : BusCreator  Inputs=12
  Bus Creator12 : BusCreator  Inputs=8
  Bus Creator13 : BusCreator  Inputs=4
  Bus Creator16 : BusCreator  Inputs=5
  Bus Creator2 : BusCreator  Inputs=28
  Bus Creator3 : BusCreator  Inputs=4
  Bus Creator9 : BusCreator  Inputs=6
  Bus Selector : BusSelector  OutputSignals=Aerodynamics_Output.fx_air,Aerodynamics_Output.fy_air,Aerodynamics_Output.fz_air,Aerodynamics_Output.mx_air,Aerodynamics_Output.my_air,Aerodynamics_Output.mz_air
  Bus Selector1 : BusSelector  OutputSignals=Suspension_States,Suspension_Kinematics,Suspension_Forces
  Bus Selector2 : BusSelector  OutputSignals=Steer_States.q0,Steer_States.q7,Steer_States.q8,Steer_States.q9,Steer_States.q10,Steer_States.u0,Steer_States.u7,Steer_States.u8,Steer_States.u9,Steer_States.u10,Steer2Body,Steer_Forces
  Bus Selector3 : BusSelector  OutputSignals=Powertrain_Output.iw_eff_pt_lf,Powertrain_Output.iw_eff_pt_rf,Powertrain_Output.iw_eff_pt_lr,Powertrain_Output.iw_eff_pt_rr,Powertrain_Output.my_drv_lf,Powertrain_Output.my_drv_rf,Powertrain_Output.my_drv_lr,Powertrain_Output.my_drv_rr
  Bus Selector4 : BusSelector  OutputSignals=Brake_Output.fm_brk_lf,Brake_Output.fm_brk_rf,Brake_Output.fm_brk_lr,Brake_Output.fm_brk_rr
  Bus Selector5 : BusSelector  OutputSignals=Tire_Forces_LF,Tire_Forces_RF,Tire_Forces_LR,Tire_Forces_RR,Tire_Forees_GND
  Bus Selector6 : BusSelector  OutputSignals=Chassi_States.q0,Chassi_States.q1,Chassi_States.q2,Chassi_States.q3,Chassi_States.q4,Chassi_States.q5,Chassi_States.u0,Chassi_States.u1,Chassi_States.u2,Chassi_States.u3,Chassi_States.u4,Chassi_States.u5,Wheel_LF.q0,Wheel_LF.q1,Wheel_LF.u0,Wheel_LF.u1,Wheel_RF.q0,Wheel_RF.q1,Wheel_RF.u0,Wheel_RF.u1,Wheel_LR.q0,Wheel_LR.q1,Wheel_LR.u0,Wheel_LR.u1,Wheel_RR.q0,Wheel_RR.q1,Wheel_RR.u0,Wheel_RR.u1
  Bus to Vector{1..11} (11 alike) : BusToVector
  Memory : Memory
  Tires : Subsystem
  body_kinematic_out_whl_lf : Subsystem
  body_kinematic_out_whl_lf1 : Subsystem
  body_kinematic_out_whl_lf2 : Subsystem
  body_kinematic_out_whl_lf3 : Subsystem
  Out1 : Outport
  Out2 : Outport  Port=2
  Out3 : Outport  Port=3
  wires:
  Bus Selector5/5 -> Bus Creator16/5  "<Tire_Forees_GND>"
  Tires/6(Tire Force Ground) -> Bus Creator1/6  "Tire_Forees_GND"
  Aero Input/1 -> Bus Selector/1
  Susp Input/1 -> Bus Selector1/1
  Body/1(State) -> Bus Creator/1  "Chassi_States"
  Body/2(Chassis) -> Bus Creator/2  "Chassis_Motion"
  Body/3(Wheel LF) -> Bus Creator/3  "Wheel_LF"
  Body/4(Wheel RF) -> Bus Creator/4  "Wheel_RF"
  Body/5(Wheel LR) -> Bus Creator/5  "Wheel_LR"
  Body/6(Wheel RR) -> Bus Creator/6  "Wheel_RR"
  Bus Selector/1 -> Bus Creator9/1  "<fx_air>"
  Bus Selector/2 -> Bus Creator9/2  "<fy_air>"
  Bus Selector/3 -> Bus Creator9/3  "<fz_air>"
  Bus Selector/4 -> Bus Creator9/4  "<mx_air>"
  Bus Selector/5 -> Bus Creator9/5  "<my_air>"
  Bus Selector/6 -> Bus Creator9/6  "<mz_air>"
  Bus Selector1/1 -> Bus Creator10/1  "<Suspension_States>"
  Bus Selector1/2 -> Bus Creator10/2  "<Suspension_Kinematics>"
  Bus Selector3/1 -> Bus Creator12/1  "<iw_eff_pt_lf>"
  Bus Selector3/2 -> Bus Creator12/2  "<iw_eff_pt_rf>"
  Bus Selector3/3 -> Bus Creator12/3  "<iw_eff_pt_lr>"
  Bus Selector3/4 -> Bus Creator12/4  "<iw_eff_pt_rr>"
  Bus Selector4/1 -> Bus Creator13/1  "<fm_brk_lf>"
  Bus Selector4/2 -> Bus Creator13/2  "<fm_brk_rf>"
  Bus Selector4/3 -> Bus Creator13/3  "<fm_brk_lr>"
  Bus Selector4/4 -> Bus Creator13/4  "<fm_brk_rr>"
  Bus Selector5/1 -> Bus Creator16/1  "<Tire_Forces_LF>"
  Bus Selector5/2 -> Bus Creator16/2  "<Tire_Forces_RF>"
  Bus Selector5/3 -> Bus Creator16/3  "<Tire_Forces_LR>"
  Bus Selector5/4 -> Bus Creator16/4  "<Tire_Forces_RR>"
  Bus Creator16/1 -> Bus to Vector6/1
  Bus Selector2/1 -> Bus Creator11/1  "<q0>"
  Bus Selector2/2 -> Bus Creator11/2  "<q7>"
  Bus Selector2/3 -> Bus Creator11/3  "<q8>"
  Bus Selector2/4 -> Bus Creator11/4  "<q9>"
  Bus Selector2/5 -> Bus Creator11/5  "<q10>"
  Bus Selector2/6 -> Bus Creator11/6  "<u0>"
  Bus Selector2/7 -> Bus Creator11/7  "<u7>"
  Bus Selector2/8 -> Bus Creator11/8  "<u8>"
  Bus Selector2/9 -> Bus Creator11/9  "<u9>"
  Bus Selector2/10 -> Bus Creator11/10  "<u10>"
  Bus Selector2/11 -> Bus Creator11/11  "<Steer2Body>"
  Bus Selector2/12 -> Bus Creator11/12  "<Steer_Forces>"
  Bus Creator/1 -> Out1/1, [VehDynBus]
  Tires/1(Tire States) -> Bus Creator1/1  "Tires_States"
  Tires/2(Tire LF) -> Bus Creator1/2  "Tire_Forces_LF"
  Tires/3(Tire RF) -> Bus Creator1/3  "Tire_Forces_RF"
  Tires/4(Tire LR) -> Bus Creator1/4  "Tire_Forces_LR"
  Tires/5(Tire RR) -> Bus Creator1/5  "Tire_Forces_RR"
  Bus Creator1/1 -> Bus Selector5/1, Out2/1  "Tires_Bus"
  Power Input/1 -> Bus Selector3/1
  Direct Input/1 -> Body/7(Direct Input)
  Brake Input/1 -> Bus Selector4/1
  Body Model/1 -> body_kinematic_out_whl_lf/1(In1)
  Body Model/2 -> body_kinematic_out_whl_lf1/1(In1)
  Body Model/3 -> body_kinematic_out_whl_lf2/1(In1)
  Body Model/4 -> body_kinematic_out_whl_lf3/1(In1)
  Steer Input/1 -> Bus Selector2/1
  Bus Selector1/3 -> Bus Creator10/3  "<Suspension_Forces>"
  Bus Selector3/5 -> Bus Creator12/5  "<my_drv_lf>"
  Bus Selector3/6 -> Bus Creator12/6  "<my_drv_rf>"
  Bus Selector3/7 -> Bus Creator12/7  "<my_drv_lr>"
  Bus Selector3/8 -> Bus Creator12/8  "<my_drv_rr>"
  Bus Creator10/1 -> Bus to Vector1/1
  [VehDynBus] -> Bus Selector6/1
  Bus Selector6/1 -> Bus Creator2/1  "<q0>"
  Bus Selector6/2 -> Bus Creator2/2  "<q1>"
  Bus Selector6/3 -> Bus Creator2/3  "<q2>"
  Bus Selector6/4 -> Bus Creator2/4  "<q3>"
  Bus Selector6/5 -> Bus Creator2/5  "<q4>"
  Bus Selector6/6 -> Bus Creator2/6  "<q5>"
  Bus Selector6/7 -> Bus Creator2/7  "<u0>"
  Bus Selector6/8 -> Bus Creator2/8  "<u1>"
  Bus Selector6/9 -> Bus Creator2/9  "<u2>"
  Bus Selector6/10 -> Bus Creator2/10  "<u3>"
  Bus Selector6/11 -> Bus Creator2/11  "<u4>"
  Bus Selector6/12 -> Bus Creator2/12  "<u5>"
  Bus Selector6/13 -> Bus Creator2/13  "<q0>"
  Bus Selector6/14 -> Bus Creator2/14  "<q1>"
  Bus Selector6/15 -> Bus Creator2/15  "<u0>"
  Bus Selector6/16 -> Bus Creator2/16  "<u1>"
  Bus Selector6/17 -> Bus Creator2/17  "<q0>"
  Bus Selector6/18 -> Bus Creator2/18  "<q1>"
  Bus Selector6/19 -> Bus Creator2/19  "<u0>"
  Bus Selector6/20 -> Bus Creator2/20  "<u1>"
  Bus Selector6/21 -> Bus Creator2/21  "<q0>"
  Bus Selector6/22 -> Bus Creator2/22  "<q1>"
  Bus Selector6/23 -> Bus Creator2/23  "<u0>"
  Bus Selector6/24 -> Bus Creator2/24  "<u1>"
  Bus Selector6/25 -> Bus Creator2/25  "<q0>"
  Bus Selector6/26 -> Bus Creator2/26  "<q1>"
  Bus Selector6/27 -> Bus Creator2/27  "<u0>"
  Bus Selector6/28 -> Bus Creator2/28  "<u1>"
  Bus Creator2/1 -> Memory/1
  Memory/1 -> Bus to Vector11/1
  Bus Creator11/1 -> Bus to Vector2/1
  Bus Creator9/1 -> Bus to Vector3/1
  Bus Creator12/1 -> Bus to Vector4/1
  Bus Creator13/1 -> Bus to Vector5/1
  body_kinematic_out_whl_lf/1(Out1) -> Bus to Vector7/1, Bus Creator3/1  "bodykin_whl_out_lf"
  body_kinematic_out_whl_lf1/1(Out1) -> Bus to Vector8/1, Bus Creator3/2  "bodykin_whl_out_rf"
  body_kinematic_out_whl_lf2/1(Out1) -> Bus to Vector9/1, Bus Creator3/3  "bodykin_whl_out_lr"
  body_kinematic_out_whl_lf3/1(Out1) -> Bus to Vector10/1, Bus Creator3/4  "bodykin_whl_out_rr"
  Bus Creator3/1 -> Out3/1  "bodykinematic_wheel_bus"
  Bus to Vector3/1 -> Body/1(Aero Input)
  Bus to Vector1/1 -> Body/2(Susp Input), Body Model/1
  Bus to Vector2/1 -> Body/3(Steer Input), Body Model/2
  Bus to Vector4/1 -> Body/4(Power Input)
  Bus to Vector5/1 -> Body/5(Brake Input)
  Bus to Vector6/1 -> Body/6(Tires Input)
  Bus to Vector7/1 -> Tires/1(Wheel LF)
  Bus to Vector8/1 -> Tires/2(Wheel RF)
  Bus to Vector9/1 -> Tires/3(Wheel LR)
  Bus to Vector10/1 -> Tires/4(Wheel RR)
  Bus to Vector11/1 -> Body Model/3

== system FCW_a1/Veh_1_1/ComplexVehicleModel/Brake ==
  Body Input : Inport
  Driver Input : Inport  Port=2
  Inertia Wheel : Inport  Port=3
  Fz Wheel : Inport  Port=4
  Direct Input : Inport  Port=5
  Brake Model : S-Function  FunctionName=panoBrake_sfun  Parameters='5aa55ff1-4ffb-47ef-b8cb-7b2ffdefc837'  SFunctionDeploymentMode=off  EnableBusSupport=off
  Brake States : Subsystem
  Memory : Memory
  SteerStates1 : Subsystem
  BrakeStates : Outport
  BrakeOutput : Outport  Port=2
  wires:
  Direct Input/1 -> Brake Model/5
  Brake Model/1 -> Brake States/1(In1)
  Brake Model/2 -> SteerStates1/1(In1)
  Body Input/1 -> Memory/1
  Driver Input/1 -> Brake Model/2
  Inertia Wheel/1 -> Brake Model/3
  Fz Wheel/1 -> Brake Model/4
  Brake States/1(Out1) -> BrakeStates/1
  SteerStates1/1(Out1) -> BrakeOutput/1
  Memory/1 -> Brake Model/1

== system FCW_a1/Veh_1_1/ComplexVehicleModel/Powertrain ==
  Body Input : Inport
  Throttle : Inport  Port=2
  TransMode : Inport  Port=3
  Gear : Inport  Port=4
  BrakeSignal : Inport  Port=5
  Memory : Memory
  Powertrain Model : S-Function  FunctionName=panoPowertrain_sfun  Parameters='5aa55ff1-4ffb-47ef-b8cb-7b2ffdefc837'  SFunctionDeploymentMode=off  EnableBusSupport=off
  PowertrainOut : Subsystem
  PowertrainStates : Subsystem
  Powertrain States : Outport
  Powertrain Output : Outport  Port=2
  wires:
  BrakeSignal/1 -> Powertrain Model/5
  Gear/1 -> Powertrain Model/4
  TransMode/1 -> Powertrain Model/3
  Throttle/1 -> Powertrain Model/2
  Powertrain Model/1 -> PowertrainStates/1(In1)
  PowertrainStates/1(Out1) -> Powertrain States/1
  PowertrainOut/1(Out1) -> Powertrain Output/1
  Powertrain Model/2 -> PowertrainOut/1(In1)
  Memory/1 -> Powertrain Model/1
  Body Input/1 -> Memory/1

== system FCW_a1/Veh_1_1/ComplexVehicleModel/Steer ==
  Body Input : Inport
  Steer Angle : Inport  Port=2
  Suspension Input : Inport  Port=3
  Tire Input : Inport  Port=4
  Direct Steer : Inport  Port=5
  Memory : Memory
  Memory1 : Memory
  SteerForces : Subsystem
  SteerKinemateics : Subsystem
  SteerStates : Subsystem
  SteerToBody : Subsystem
  Steering Model : S-Function  FunctionName=panoSteer_sfun  Parameters='5aa55ff1-4ffb-47ef-b8cb-7b2ffdefc837'  SFunctionDeploymentMode=off  EnableBusSupport=off
  Steer States : Outport
  Steer Kinematiocs : Outport  Port=2
  Steer2Body : Outport  Port=3
  Steer Forces : Outport  Port=4
  wires:
  Direct Steer/1 -> Steering Model/5
  Body Input/1 -> Memory/1
  Suspension Input/1 -> Steering Model/3
  Tire Input/1 -> Memory1/1
  Steer Angle/1 -> Steering Model/2
  Steering Model/1 -> SteerStates/1(In1)
  SteerStates/1(Out1) -> Steer States/1  "Steer_States"
  SteerKinemateics/1(Out1) -> Steer Kinematiocs/1  "Steer_Kinematics"
  SteerToBody/1(Out1) -> Steer2Body/1  "SteertoBody"
  SteerForces/1(Out1) -> Steer Forces/1  "Steer_Forces"
  Steering Model/2 -> SteerKinemateics/1(In1)
  Steering Model/3 -> SteerToBody/1(In1)
  Steering Model/4 -> SteerForces/1(In1)
  Memory/1 -> Steering Model/1
  Memory1/1 -> Steering Model/4

== system FCW_a1/Veh_1_1/ComplexVehicleModel/Suspensions ==
  Body Input : Inport
  WheelLF Input : Inport  Port=2
  WheelRF Input : Inport  Port=3
  WheelLR Input : Inport  Port=4
  WheelRR Input : Inport  Port=5
  Memory{,1..4} (5 alike) : Memory
  SupensionsStates : Subsystem
  Suspension Model : S-Function  FunctionName=panoSuspension_sfun  Parameters='5aa55ff1-4ffb-47ef-b8cb-7b2ffdefc837'  SFunctionDeploymentMode=off  EnableBusSupport=off
  SuspensionForces : Subsystem
  SuspensionKinematics : Subsystem
  SuspensionSteer : Subsystem
  Suspensions States : Outport
  Suspension Kinematics : Outport  Port=2
  Suspension Forces : Outport  Port=3
  Suspension Steer : Outport  Port=4
  wires:
  Body Input/1 -> Memory/1
  WheelLF Input/1 -> Memory1/1
  WheelRF Input/1 -> Memory2/1
  WheelLR Input/1 -> Memory3/1
  WheelRR Input/1 -> Memory4/1
  Suspension Model/1 -> SupensionsStates/1(In1)
  SupensionsStates/1(Out1) -> Suspensions States/1  "Supension_States"
  SuspensionKinematics/1(Out1) -> Suspension Kinematics/1  "Suspension_Kinematics"
  SuspensionForces/1(Out1) -> Suspension Forces/1  "Suspension_Forces"
  SuspensionSteer/1(Out1) -> Suspension Steer/1  "Suspension_Steer"
  Suspension Model/2 -> SuspensionKinematics/1(In1)
  Suspension Model/3 -> SuspensionForces/1(In1)
  Suspension Model/4 -> SuspensionSteer/1(In1)
  Memory/1 -> Suspension Model/1
  Memory1/1 -> Suspension Model/2
  Memory2/1 -> Suspension Model/3
  Memory3/1 -> Suspension Model/4
  Memory4/1 -> Suspension Model/5

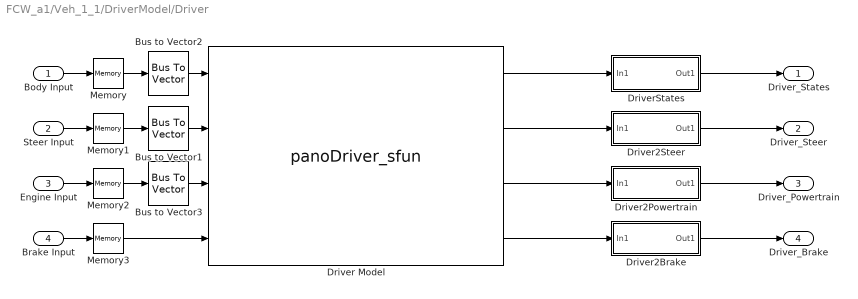
== system FCW_a1/Veh_1_1/DriverModel/Driver ==
  Body Input : Inport
  Steer Input : Inport  Port=2
  Engine Input : Inport  Port=3
  Brake Input : Inport  Port=4
  Bus to Vector1 : BusToVector
  Bus to Vector2 : BusToVector
  Bus to Vector3 : BusToVector
  Driver Model : S-Function  FunctionName=panoDriver_sfun  Parameters='5aa55ff1-4ffb-47ef-b8cb-7b2ffdefc837'  SFunctionDeploymentMode=off  EnableBusSupport=off
  Driver2Brake : Subsystem
  Driver2Powertrain : Subsystem
  Driver2Steer : Subsystem
  DriverStates : Subsystem
  Memory{,1..3} (4 alike) : Memory
  Driver_States : Outport
  Driver_Steer : Outport  Port=2
  Driver_Powertrain : Outport  Port=3
  Driver_Brake : Outport  Port=4
  wires:
  Memory3/1 -> Driver Model/4
  Memory2/1 -> Bus to Vector3/1
  Memory1/1 -> Bus to Vector1/1
  Memory/1 -> Bus to Vector2/1
  Body Input/1 -> Memory/1
  Steer Input/1 -> Memory1/1
  Driver2Powertrain/1(Out1) -> Driver_Powertrain/1
  Driver2Brake/1(Out1) -> Driver_Brake/1
  Driver Model/4 -> Driver2Brake/1(In1)
  Driver Model/3 -> Driver2Powertrain/1(In1)
  Driver2Steer/1(Out1) -> Driver_Steer/1
  Driver Model/2 -> Driver2Steer/1(In1)
  DriverStates/1(Out1) -> Driver_States/1
  Driver Model/1 -> DriverStates/1(In1)
  Engine Input/1 -> Memory2/1
  Brake Input/1 -> Memory3/1
  Bus to Vector2/1 -> Driver Model/1
  Bus to Vector1/1 -> Driver Model/2
  Bus to Vector3/1 -> Driver Model/3

== system FCW_a1/Veh_1_1/Veh_1_1_Sensors/OBU_BSM ==
  In1 : Inport
  Bus : BusCreator  Inputs=20
  GeneralSensor : S-Function  FunctionName=GeneralSensorModel  Parameters='PanoDataModel.Sensor.OBU.BSM.Output','125cf20f-ac34-4e68-95de-7d1873d67c03','pos.lat@f,pos.long@f,secMark@i,accuracy.pos@f,transmission@f,speed@f,heading@i,accelSet.long@f,accelSet.lat@f,accelSet.vert@f,accelSet.yaw@f,brakes.traction@i,brakes.abs@i,brakes.scs@i,size.width@f,size.length@f,vehicleClass.classification@i,safetyExt.events@i,safetyExt.lights@i','10.00','64'  SFunctionDeploymentMode=off  EnableBusSupport=off
  Out1 : Outport
  wires:
  GeneralSensor/1 -> Bus/1  "Width"
  In1/1 -> GeneralSensor/1
  Bus/1 -> Out1/1
  GeneralSensor/2 -> Bus/2  "pos.lat"
  GeneralSensor/3 -> Bus/3  "pos.long"
  GeneralSensor/4 -> Bus/4  "secMark"
  GeneralSensor/5 -> Bus/5  "accuracy.pos"
  GeneralSensor/6 -> Bus/6  "transmission"
  GeneralSensor/7 -> Bus/7  "speed"
  GeneralSensor/8 -> Bus/8  "heading"
  GeneralSensor/9 -> Bus/9  "accelSet.long"
  GeneralSensor/10 -> Bus/10  "accelSet.lat"
  GeneralSensor/11 -> Bus/11  "accelSet.vert"
  GeneralSensor/12 -> Bus/12  "accelSet.yaw"
  GeneralSensor/13 -> Bus/13  "brakes.traction"
  GeneralSensor/14 -> Bus/14  "brakes.abs"
  GeneralSensor/15 -> Bus/15  "brakes.scs"
  GeneralSensor/16 -> Bus/16  "size.width"
  GeneralSensor/17 -> Bus/17  "size.length"
  GeneralSensor/18 -> Bus/18  "vehicleClass.classification"
  GeneralSensor/19 -> Bus/19  "safetyExt.events"
  GeneralSensor/20 -> Bus/20  "safetyExt.lights"

== system FCW_a1/Veh_1/ComplexVehicleModel/Aerodynamics/Chassis States ==
  In1 : Inport
  Bus Creator : BusCreator  Inputs=12
  Demux : Demux  Outputs=12
  Out1 : Outport
  wires:
  In1/1 -> Demux/1
  Demux/1 -> Bus Creator/1  "beta_air"
  Demux/2 -> Bus Creator/2  "pitch_air"
  Demux/3 -> Bus Creator/3  "yawwind_air"
  Demux/4 -> Bus Creator/4  "v_air"
  Demux/5 -> Bus Creator/5  "vwind_air"
  Demux/6 -> Bus Creator/6  "z_air"
  Demux/7 -> Bus Creator/7  "fx_air"
  Demux/8 -> Bus Creator/8  "fy_air"
  Demux/9 -> Bus Creator/9  "fz_air"
  Demux/10 -> Bus Creator/10  "mx_air"
  Demux/11 -> Bus Creator/11  "my_air"
  Demux/12 -> Bus Creator/12  "mz_air"
  Bus Creator/1 -> Out1/1  "Aerodynamics_States"

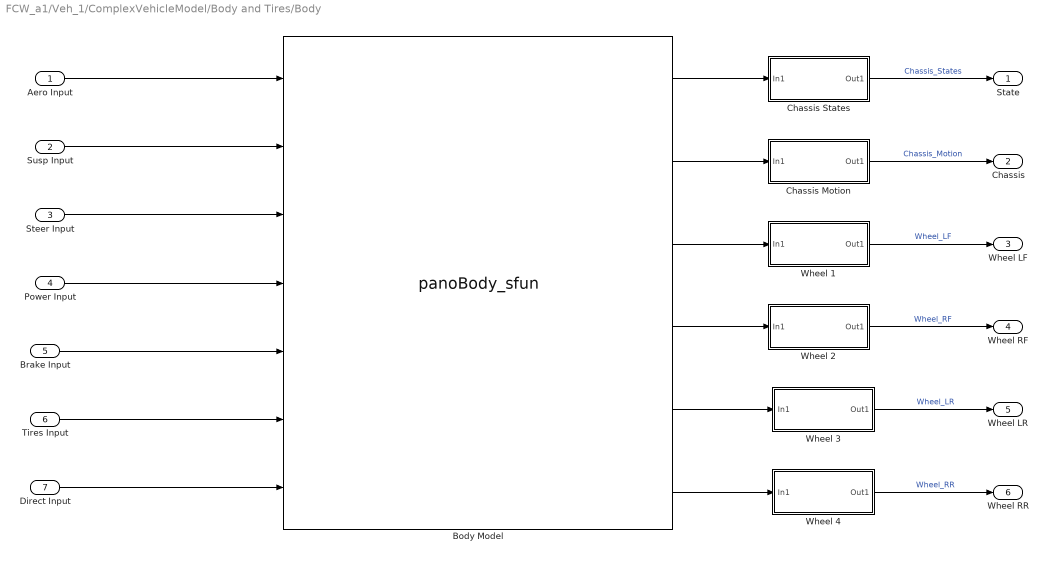
== system FCW_a1/Veh_1/ComplexVehicleModel/Body and Tires/Body ==
  Aero Input : Inport
  Susp Input : Inport  Port=2
  Steer Input : Inport  Port=3
  Power Input : Inport  Port=4
  Brake Input : Inport  Port=5
  Tires Input : Inport  Port=6
  Direct Input : Inport  Port=7
  Body Model : S-Function  FunctionName=panoBody_sfun  Parameters='2f869580-59bc-4052-87af-10578d1ae191'  SFunctionDeploymentMode=off  EnableBusSupport=off
  Chassis Motion : Subsystem
  Chassis States : Subsystem
  Wheel 1 : Subsystem
  Wheel 2 : Subsystem
  Wheel 3 : Subsystem
  Wheel 4 : Subsystem
  State : Outport
  Chassis : Outport  Port=2
  Wheel LF : Outport  Port=3
  Wheel RF : Outport  Port=4
  Wheel LR : Outport  Port=5
  Wheel RR : Outport  Port=6
  wires:
  Direct Input/1 -> Body Model/7
  Body Model/2 -> Chassis Motion/1(In1)
  Chassis Motion/1(Out1) -> Chassis/1  "Chassis_Motion"
  Body Model/1 -> Chassis States/1(In1)
  Chassis States/1(Out1) -> State/1  "Chassis_States"
  Body Model/3 -> Wheel 1/1(In1)
  Wheel 1/1(Out1) -> Wheel LF/1  "Wheel_LF"
  Body Model/4 -> Wheel 2/1(In1)
  Body Model/5 -> Wheel 3/1(In1)
  Body Model/6 -> Wheel 4/1(In1)
  Wheel 3/1(Out1) -> Wheel LR/1  "Wheel_LR"
  Wheel 4/1(Out1) -> Wheel RR/1  "Wheel_RR"
  Wheel 2/1(Out1) -> Wheel RF/1  "Wheel_RF"
  Tires Input/1 -> Body Model/6
  Power Input/1 -> Body Model/4
  Brake Input/1 -> Body Model/5
  Steer Input/1 -> Body Model/3
  Susp Input/1 -> Body Model/2
  Aero Input/1 -> Body Model/1

== system FCW_a1/Veh_1/ComplexVehicleModel/Body and Tires/Tires ==
  Wheel LF : Inport
  Wheel RF : Inport  Port=2
  Wheel LR : Inport  Port=3
  Wheel RR : Inport  Port=4
  Tires Force  2 : Subsystem
  "Tires Force 1 " : Subsystem
  Tires Force 3 : Subsystem
  Tires Force 4 : Subsystem
  Tires Force Ground : Subsystem
  Tires Model : S-Function  FunctionName=panoTire_sfun  Parameters='2f869580-59bc-4052-87af-10578d1ae191'  SFunctionDeploymentMode=off  EnableBusSupport=off
  TiresStates : Subsystem
  Tire States : Outport
  Tire LF : Outport  Port=2
  Tire RF : Outport  Port=3
  Tire LR : Outport  Port=4
  Tire RR : Outport  Port=5
  Tire Force Ground : Outport  Port=6
  wires:
  Tires Model/6 -> Tires Force Ground/1(In1)
  Tires Force Ground/1(Out1) -> Tire Force Ground/1  "Tire_Forces_GND"
  Wheel LF/1 -> Tires Model/1
  Wheel RF/1 -> Tires Model/2
  Wheel LR/1 -> Tires Model/3
  Wheel RR/1 -> Tires Model/4
  Tires Model/1 -> TiresStates/1(In1)
  TiresStates/1(Out1) -> Tire States/1  "Tires_States"
  Tires Model/2 -> "Tires Force 1 "/1(In1)
  "Tires Force 1 "/1(Out1) -> Tire LF/1  "Tire_Forces_LF"
  Tires Model/5 -> Tires Force 4/1(In1)
  Tires Model/4 -> Tires Force 3/1(In1)
  Tires Model/3 -> Tires Force  2/1(In1)
  Tires Force 3/1(Out1) -> Tire LR/1  "Tire_Forces_LR"
  Tires Force 4/1(Out1) -> Tire RR/1  "Tire_Forces_RR"
  Tires Force  2/1(Out1) -> Tire RF/1  "Tire_Forces_RF"

== system FCW_a1/Veh_1/ComplexVehicleModel/Body and Tires/body_kinematic_out_whl_lf ==
  In1 : Inport
  Bus Creator : BusCreator  Inputs=18
  Demux : Demux  Outputs=18
  Out1 : Outport
  wires:
  In1/1 -> Demux/1
  Demux/1 -> Bus Creator/1  "rot_whl"
  Demux/2 -> Bus Creator/2  "w_whl"
  Demux/3 -> Bus Creator/3  "z_whl_whl"
  Demux/4 -> Bus Creator/4  "yaw_whl"
  Demux/5 -> Bus Creator/5  "pitch_whl"
  Demux/6 -> Bus Creator/6  "roll_whl"
  Demux/7 -> Bus Creator/7  "vwx_whl"
  Demux/8 -> Bus Creator/8  "vwy_whl"
  Demux/9 -> Bus Creator/9  "vwz_whl"
  Demux/10 -> Bus Creator/10  "avwx_whl"
  Demux/11 -> Bus Creator/11  "avwy_whl"
  Demux/12 -> Bus Creator/12  "avwz_whl"
  Demux/13 -> Bus Creator/13  "dzdx_whl"
  Demux/14 -> Bus Creator/14  "dzdy_whl"
  Demux/15 -> Bus Creator/15  "xgnd_whl"
  Demux/16 -> Bus Creator/16  "ygnd_whl"
  Demux/17 -> Bus Creator/17  "zgnd_whl"
  Demux/18 -> Bus Creator/18  "mux_whl"
  Bus Creator/1 -> Out1/1  "bodykin_whl_out"

== system FCW_a1/Veh_1/ComplexVehicleModel/Body and Tires/body_kinematic_out_whl_lf1 ==
  In1 : Inport
  Bus Creator : BusCreator  Inputs=18
  Demux : Demux  Outputs=18
  Out1 : Outport
  wires:
  Bus Creator/1 -> Out1/1  "bodykin_whl_out"
  Demux/18 -> Bus Creator/18  "mux_whl"
  Demux/17 -> Bus Creator/17  "zgnd_whl"
  Demux/16 -> Bus Creator/16  "ygnd_whl"
  Demux/15 -> Bus Creator/15  "xgnd_whl"
  Demux/14 -> Bus Creator/14  "dzdy_whl"
  Demux/13 -> Bus Creator/13  "dzdx_whl"
  Demux/12 -> Bus Creator/12  "avwz_whl"
  Demux/11 -> Bus Creator/11  "avwy_whl"
  Demux/10 -> Bus Creator/10  "avwx_whl"
  Demux/9 -> Bus Creator/9  "vwz_whl"
  Demux/8 -> Bus Creator/8  "vwy_whl"
  Demux/7 -> Bus Creator/7  "vwx_whl"
  Demux/6 -> Bus Creator/6  "roll_whl"
  Demux/5 -> Bus Creator/5  "pitch_whl"
  Demux/4 -> Bus Creator/4  "yaw_whl"
  Demux/3 -> Bus Creator/3  "z_whl_whl"
  Demux/2 -> Bus Creator/2  "w_whl"
  Demux/1 -> Bus Creator/1  "rot_whl"
  In1/1 -> Demux/1
